simulink model "Simulink_asserv_Disc_5Avril_V2023a"  (R2023a)
settings: Solver=ode45  StartTime=0.0  StopTime=2500  FixedStep=0.01  RelTol=1e-3
model workspace (MAT data in the model file):
  AmbiantTemp = Simulink.Parameter
  AmbiantTemp.Value = 23
  AmbiantTemp.DataType = 'auto'
  AmbiantTemp.Complexity = 'real'
  AmbiantTemp.Dimensions = [1 1]
  CondSig_mesureTemp_Gain = Simulink.Parameter
  CondSig_mesureTemp_Gain.Value = 3.3
  CondSig_mesureTemp_Gain.DataType = 'auto'
  CondSig_mesureTemp_Gain.Complexity = 'real'
  CondSig_mesureTemp_Gain.Dimensions = [1 1]
  CondSig_mesureTemp_Vsub = Simulink.Parameter
  CondSig_mesureTemp_Vsub.Value = 1.85
  CondSig_mesureTemp_Vsub.DataType = 'auto'
  CondSig_mesureTemp_Vsub.Complexity = 'real'
  CondSig_mesureTemp_Vsub.Dimensions = [1 1]
  Consigne1_Temps = Simulink.Parameter
  Consigne1_Temps.Value = 640
  Consigne1_Temps.DataType = 'auto'
  Consigne1_Temps.Complexity = 'real'
  Consigne1_Temps.Dimensions = [1 1]
  Consigne1_Valeur = Simulink.Parameter
  Consigne1_Valeur.Value = 30
  Consigne1_Valeur.DataType = 'auto'
  Consigne1_Valeur.Complexity = 'real'
  Consigne1_Valeur.Dimensions = [1 1]
  Consigne2_Temps = Simulink.Parameter
  Consigne2_Temps.Value = 1290
  Consigne2_Temps.DataType = 'auto'
  Consigne2_Temps.Complexity = 'real'
  Consigne2_Temps.Dimensions = [1 1]
  Consigne2_Valeur = Simulink.Parameter
  Consigne2_Valeur.Value = 20
  Consigne2_Valeur.DataType = 'auto'
  Consigne2_Valeur.Complexity = 'real'
  Consigne2_Valeur.Dimensions = [1 1]
  Consigne3_Temps = Simulink.Parameter
  Consigne3_Temps.Value = 2130
  Consigne3_Temps.DataType = 'auto'
  Consigne3_Temps.Complexity = 'real'
  Consigne3_Temps.Dimensions = [1 1]
  Consigne3_Valeur = Simulink.Parameter
  Consigne3_Valeur.Value = 25
  Consigne3_Valeur.DataType = 'auto'
  Consigne3_Valeur.Complexity = 'real'
  Consigne3_Valeur.Dimensions = [1 1]
  DivTen_mesureTemp_R_pullup = Simulink.Parameter
  DivTen_mesureTemp_R_pullup.Value = 10000
  DivTen_mesureTemp_R_pullup.DataType = 'auto'
  DivTen_mesureTemp_R_pullup.Complexity = 'real'
  DivTen_mesureTemp_R_pullup.Dimensions = [1 1]
  DivTen_mesureTemp_Vcc = Simulink.Parameter
  DivTen_mesureTemp_Vcc.Value = 5
  DivTen_mesureTemp_Vcc.DataType = 'auto'
  DivTen_mesureTemp_Vcc.Complexity = 'real'
  DivTen_mesureTemp_Vcc.Dimensions = [1 1]
  Gain_Comparateur_VoltageControle = Simulink.Parameter
  Gain_Comparateur_VoltageControle.Value = 0.32
  Gain_Comparateur_VoltageControle.DataType = 'auto'
  Gain_Comparateur_VoltageControle.Complexity = 'real'
  Gain_Comparateur_VoltageControle.Dimensions = [1 1]
  GuT1_Denominateur = Simulink.Parameter
  GuT1_Denominateur.Value = [83.71 1]
  GuT1_Denominateur.DataType = 'auto'
  GuT1_Denominateur.Complexity = 'real'
  GuT1_Denominateur.Dimensions = [1 2]
  GuT1_Numerateur = Simulink.Parameter
  GuT1_Numerateur.Value = 9.96
  GuT1_Numerateur.DataType = 'auto'
  GuT1_Numerateur.Complexity = 'real'
  GuT1_Numerateur.Dimensions = [1 1]
  GuT2_Denominateur = Simulink.Parameter
  GuT2_Denominateur.Value = [909.26 121.79 1]
  GuT2_Denominateur.DataType = 'auto'
  GuT2_Denominateur.Complexity = 'real'
  GuT2_Denominateur.Dimensions = [1 3]
  GuT2_Numerateur = Simulink.Parameter
  GuT2_Numerateur.Value = 8.07
  GuT2_Numerateur.DataType = 'auto'
  GuT2_Numerateur.Complexity = 'real'
  GuT2_Numerateur.Dimensions = [1 1]
  GuT3_Denominateur = Simulink.Parameter
  GuT3_Denominateur.Value = [2602.39 136.94 1]
  GuT3_Denominateur.DataType = 'auto'
  GuT3_Denominateur.Complexity = 'real'
  GuT3_Denominateur.Dimensions = [1 3]
  GuT3_Numerateur = Simulink.Parameter
  GuT3_Numerateur.Value = 7.09
  GuT3_Numerateur.DataType = 'auto'
  GuT3_Numerateur.Complexity = 'real'
  GuT3_Numerateur.Dimensions = [1 1]
  Nombre_bits_ADC = Simulink.Parameter
  Nombre_bits_ADC.Value = 10
  Nombre_bits_ADC.DataType = 'auto'
  Nombre_bits_ADC.Complexity = 'real'
  Nombre_bits_ADC.Dimensions = [1 1]
  Nombre_bits_DAC = Simulink.Parameter
  Nombre_bits_DAC.Value = 8
  Nombre_bits_DAC.DataType = 'auto'
  Nombre_bits_DAC.Complexity = 'real'
  Nombre_bits_DAC.Dimensions = [1 1]
  PerturbT1_Denominateur = Simulink.Parameter
  PerturbT1_Denominateur.Value = [127 1]
  PerturbT1_Denominateur.DataType = 'auto'
  PerturbT1_Denominateur.Complexity = 'real'
  PerturbT1_Denominateur.Dimensions = [1 2]
  PerturbT1_Numerateur = Simulink.Parameter
  PerturbT1_Numerateur.Value = 20.9
  PerturbT1_Numerateur.DataType = 'auto'
  PerturbT1_Numerateur.Complexity = 'real'
  PerturbT1_Numerateur.Dimensions = [1 1]
  PerturbT2_Denominateur = Simulink.Parameter
  PerturbT2_Denominateur.Value = [144 1]
  PerturbT2_Denominateur.DataType = 'auto'
  PerturbT2_Denominateur.Complexity = 'real'
  PerturbT2_Denominateur.Dimensions = [1 2]
  PerturbT2_Numerateur = Simulink.Parameter
  PerturbT2_Numerateur.Value = 22
  PerturbT2_Numerateur.DataType = 'auto'
  PerturbT2_Numerateur.Complexity = 'real'
  PerturbT2_Numerateur.Dimensions = [1 1]
  PerturbT3_Denominateur = Simulink.Parameter
  PerturbT3_Denominateur.Value = [3300 167 1]
  PerturbT3_Denominateur.DataType = 'auto'
  PerturbT3_Denominateur.Complexity = 'real'
  PerturbT3_Denominateur.Dimensions = [1 3]
  PerturbT3_Numerateur = Simulink.Parameter
  PerturbT3_Numerateur.Value = 18.7
  PerturbT3_Numerateur.DataType = 'auto'
  PerturbT3_Numerateur.Complexity = 'real'
  PerturbT3_Numerateur.Dimensions = [1 1]
  Perturbation_Resistance = Simulink.Parameter
  Perturbation_Resistance.Value = 25
  Perturbation_Resistance.DataType = 'auto'
  Perturbation_Resistance.Complexity = 'real'
  Perturbation_Resistance.Dimensions = [1 1]
  Perturbation_TempsApplication = Simulink.Parameter
  Perturbation_TempsApplication.Value = 100
  Perturbation_TempsApplication.DataType = 'auto'
  Perturbation_TempsApplication.Complexity = 'real'
  Perturbation_TempsApplication.Dimensions = [1 1]
  Perturbation_Tension = Simulink.Parameter
  Perturbation_Tension.Value = 5
  Perturbation_Tension.DataType = 'auto'
  Perturbation_Tension.Complexity = 'real'
  Perturbation_Tension.Dimensions = [1 1]
  RC_deno = Simulink.Parameter
  RC_deno.Value = [3.22e-08 3.04e-05 0.00955 1]
  RC_deno.DataType = 'auto'
  RC_deno.Complexity = 'real'
  RC_deno.Dimensions = [1 4]
  Regulateur_Denominateur = Simulink.Parameter
  Regulateur_Denominateur.Value = [1 -1.913 0.913]
  Regulateur_Denominateur.DataType = 'auto'
  Regulateur_Denominateur.Complexity = 'real'
  Regulateur_Denominateur.Dimensions = [1 3]
  Regulateur_Numerateur = Simulink.Parameter
  Regulateur_Numerateur.Value = [1 -1.8995 0.901]
  Regulateur_Numerateur.DataType = 'auto'
  Regulateur_Numerateur.Complexity = 'real'
  Regulateur_Numerateur.Dimensions = [1 3]
  SourceCourant_Gain_Vcontrole_vers_A = Simulink.Parameter
  SourceCourant_Gain_Vcontrole_vers_A.Value = 3.1564
  SourceCourant_Gain_Vcontrole_vers_A.DataType = 'auto'
  SourceCourant_Gain_Vcontrole_vers_A.Complexity = 'real'
  SourceCourant_Gain_Vcontrole_vers_A.Dimensions = [1 1]
  T1T3_Denominateur = Simulink.Parameter
  T1T3_Denominateur.Value = [1 -1.9517 0.9522]
  T1T3_Denominateur.DataType = 'auto'
  T1T3_Denominateur.Complexity = 'real'
  T1T3_Denominateur.Dimensions = [1 3]
  T1T3_Numerateur = Simulink.Parameter
  T1T3_Numerateur.Value = [0 0.00019425 0.00019111]
  T1T3_Numerateur.DataType = 'auto'
  T1T3_Numerateur.Complexity = 'real'
  T1T3_Numerateur.Dimensions = [1 3]
  T2T3_Denominateur = Simulink.Parameter
  T2T3_Denominateur.Value = [1 -0.9655]
  T2T3_Denominateur.DataType = 'auto'
  T2T3_Denominateur.Complexity = 'real'
  T2T3_Denominateur.Dimensions = [1 2]
  T2T3_Numerateur = Simulink.Parameter
  T2T3_Numerateur.Value = [0 0.0303]
  T2T3_Numerateur.DataType = 'auto'
  T2T3_Numerateur.Complexity = 'real'
  T2T3_Numerateur.Dimensions = [1 2]
  ThermoRes_SHTEMP_A = Simulink.Parameter
  ThermoRes_SHTEMP_A.Value = 0.003354
  ThermoRes_SHTEMP_A.DataType = 'auto'
  ThermoRes_SHTEMP_A.Complexity = 'real'
  ThermoRes_SHTEMP_A.Dimensions = [1 1]
  ThermoRes_SHTEMP_B = Simulink.Parameter
  ThermoRes_SHTEMP_B.Value = 0.00026
  ThermoRes_SHTEMP_B.DataType = 'auto'
  ThermoRes_SHTEMP_B.Complexity = 'real'
  ThermoRes_SHTEMP_B.Dimensions = [1 1]
  ThermoRes_SHTEMP_C = Simulink.Parameter
  ThermoRes_SHTEMP_C.Value = 1.6e-06
  ThermoRes_SHTEMP_C.DataType = 'auto'
  ThermoRes_SHTEMP_C.Complexity = 'real'
  ThermoRes_SHTEMP_C.Dimensions = [1 1]
  ThermoRes_SHTEMP_D = Simulink.Parameter
  ThermoRes_SHTEMP_D.Value = 6.3e-08
  ThermoRes_SHTEMP_D.DataType = 'auto'
  ThermoRes_SHTEMP_D.Complexity = 'real'
  ThermoRes_SHTEMP_D.Dimensions = [1 1]
  ThermoRes_SH_A = Simulink.Parameter
  ThermoRes_SH_A.Value = -14.65719
  ThermoRes_SH_A.DataType = 'auto'
  ThermoRes_SH_A.Complexity = 'real'
  ThermoRes_SH_A.Dimensions = [1 1]
  ThermoRes_SH_B = Simulink.Parameter
  ThermoRes_SH_B.Value = 4798.842
  ThermoRes_SH_B.DataType = 'auto'
  ThermoRes_SH_B.Complexity = 'real'
  ThermoRes_SH_B.Dimensions = [1 1]
  ThermoRes_SH_C = Simulink.Parameter
  ThermoRes_SH_C.Value = -115334
  ThermoRes_SH_C.DataType = 'auto'
  ThermoRes_SH_C.Complexity = 'real'
  ThermoRes_SH_C.Dimensions = [1 1]
  ThermoRes_SH_D = Simulink.Parameter
  ThermoRes_SH_D.Value = -3730535
  ThermoRes_SH_D.DataType = 'auto'
  ThermoRes_SH_D.Complexity = 'real'
  ThermoRes_SH_D.Dimensions = [1 1]
  ThermoRes_SH_R_nom = Simulink.Parameter
  ThermoRes_SH_R_nom.Value = 10000
  ThermoRes_SH_R_nom.DataType = 'auto'
  ThermoRes_SH_R_nom.Complexity = 'real'
  ThermoRes_SH_R_nom.Dimensions = [1 1]
  periodeEchant = Simulink.Parameter
  periodeEchant.Value = 2
  periodeEchant.DataType = 'auto'
  periodeEchant.Complexity = 'real'
  periodeEchant.Dimensions = [1 1]
  periodeEchant_temp = Simulink.Parameter
  periodeEchant_temp.Value = 0.5
  periodeEchant_temp.DataType = 'auto'
  periodeEchant_temp.Complexity = 'real'
  periodeEchant_temp.Dimensions = [1 1]
  setupDelay = Simulink.Parameter
  setupDelay.Value = 4
  setupDelay.DataType = 'auto'
  setupDelay.Complexity = 'real'
  setupDelay.Dimensions = [1 1]
libraries: simulink x1
settings Model: SimulationMode=rapid-accelerator  ParameterArgumentNames=Perturbation_Resistance  Creator=alcot161  LastModifiedBy=alcot161
settings RTWCC: GPUComputeCapability=5.0

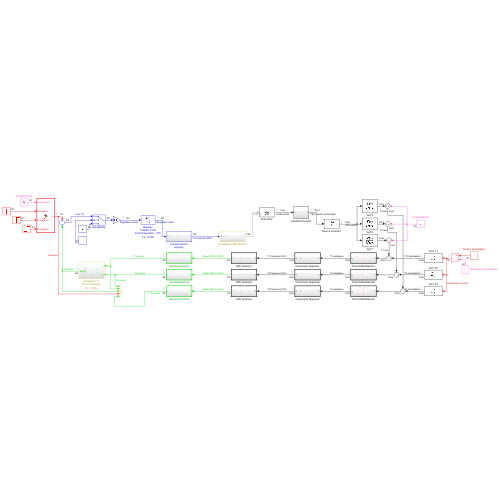
[thumbnail: Simulink's stored preview of the top-level diagram]
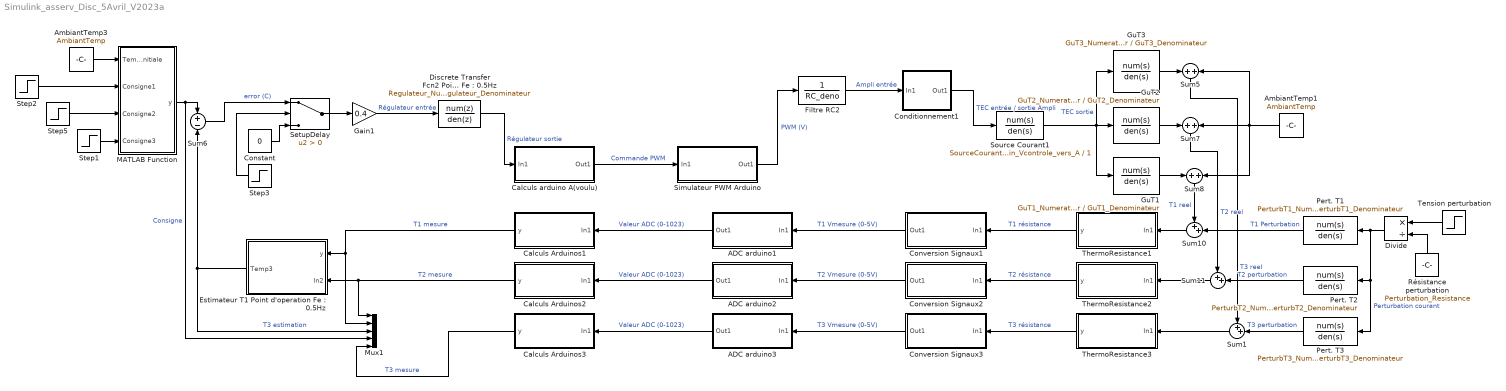
== system Simulink_asserv_Disc_5Avril_V2023a ==
  ADC arduino1 : Subsystem  TreatAsAtomicUnit=on
  ADC arduino2 : Subsystem  TreatAsAtomicUnit=on
  ADC arduino3 : Subsystem  TreatAsAtomicUnit=on
  AmbiantTemp1 : Constant  Value=AmbiantTemp
  AmbiantTemp3 : Constant  Value=AmbiantTemp
  Calculs Arduinos1 : Subsystem  TreatAsAtomicUnit=on
  Calculs Arduinos2 : Subsystem  TreatAsAtomicUnit=on
  Calculs Arduinos3 : Subsystem  TreatAsAtomicUnit=on
  "Calculs arduino A(voulu) " : Subsystem
  Conditionnement1 : Subsystem
  Constant : Constant  Value=0  SampleTime=periodeEchant
  Conversion Signaux1 : Subsystem  TreatAsAtomicUnit=on
  Conversion Signaux2 : Subsystem  TreatAsAtomicUnit=on
  Conversion Signaux3 : Subsystem  TreatAsAtomicUnit=on
  "Discrete Transfer Fcn2 Point d'operation : 27C Fe : 0.5Hz" : DiscreteTransferFcn  Numerator=Regulateur_Numerateur  Denominator=Regulateur_Denominateur
  Divide : Product  Inputs=*/
  "Estimateur T1 Point d'operation Fe : 0.5Hz" : Subsystem
  Filtre RC2 : TransferFcn  Denominator=RC_deno
  Gain1 : Gain  Gain=0.4
  GuT1 : TransferFcn  Numerator=GuT1_Numerateur  Denominator=GuT1_Denominateur
  GuT2 : TransferFcn  Numerator=GuT2_Numerateur  Denominator=GuT2_Denominateur
  GuT3 : TransferFcn  Numerator=GuT3_Numerateur  Denominator=GuT3_Denominateur
  MATLAB Function : MATLAB Function  TreatAsAtomicUnit=on
  Mux1 : Mux  Inputs=5
  Pert. T1 : TransferFcn  Numerator=PerturbT1_Numerateur  Denominator=PerturbT1_Denominateur
  Pert. T2 : TransferFcn  Numerator=PerturbT2_Numerateur  Denominator=PerturbT2_Denominateur
  Pert. T3 : TransferFcn  Numerator=PerturbT3_Numerateur  Denominator=PerturbT3_Denominateur
  Résistance perturbation : Constant  Value=Perturbation_Resistance
  SetupDelay : Switch  Criteria=u2 > Threshold  SaturateOnIntegerOverflow=off  InputSameDT=off
  Simulateur PWM Arduino : Subsystem
  Source Courant1 : TransferFcn  Numerator=SourceCourant_Gain_Vcontrole_vers_A  Denominator=1
  Step1 : Step  Time=Consigne3_Temps  After=Consigne3_Valeur  SampleTime=0.05
  Step2 : Step  Time=Consigne1_Temps  After=Consigne1_Valeur  SampleTime=0.05
  Step3 : Step  Time=setupDelay+1  SampleTime=periodeEchant
  Step5 : Step  Time=Consigne2_Temps  After=Consigne2_Valeur  SampleTime=0.05
  Sum1 : Sum  Inputs=++|
  Sum10 : Sum  Inputs=++|
  Sum11 : Sum  Inputs=++|
  Sum5 : Sum  Inputs=+|+
  Sum6 : Sum  Inputs=+|-  SampleTime=periodeEchant
  Sum7 : Sum  Inputs=+|+
  Sum8 : Sum  Inputs=+|+
  Tension perturbation : Step  Time=Perturbation_TempsApplication  After=Perturbation_Tension  SampleTime=0.05
  ThermoResistance1 : Subsystem  TreatAsAtomicUnit=on
  ThermoResistance2 : Subsystem  TreatAsAtomicUnit=on
  ThermoResistance3 : Subsystem  TreatAsAtomicUnit=on
  wires:
  ThermoResistance2/1(y) -> Conversion Signaux2/1(In1)  "T2 résistance"
  GuT2/1 -> Sum7/1
  Conversion Signaux2/1(Out1) -> ADC arduino2/1(In1)  "T2 Vmesure (0-5V)"
  ADC arduino2/1(Out1) -> Calculs Arduinos2/1(In1)  "Valeur ADC (0-1023)"
  Simulateur PWM Arduino/1(Out1) -> Filtre RC2/1  "PWM (V)"
  Step5/1 -> MATLAB Function/3(Consigne2)
  Conversion Signaux1/1(Out1) -> ADC arduino1/1(In1)  "T1 Vmesure (0-5V)"
  AmbiantTemp1/1 -> Sum5/2, Sum8/2, Sum7/2
  Filtre RC2/1 -> Conditionnement1/1(In1)  "Ampli entrée"
  Calculs Arduinos1/1(y) -> Mux1/2, "Estimateur T1 Point d'operation Fe : 0.5Hz"/1(y)  "T1 mesure"
  ADC arduino1/1(Out1) -> Calculs Arduinos1/1(In1)  "Valeur ADC (0-1023)"
  "Calculs arduino A(voulu) "/1(Out1) -> Simulateur PWM Arduino/1(In1)  "Commande PWM"
  Calculs Arduinos2/1(y) -> "Estimateur T1 Point d'operation Fe : 0.5Hz"/2(In2), Mux1/1  "T2 mesure"
  Source Courant1/1 -> GuT3/1, GuT1/1, GuT2/1  "TEC sortie"
  ThermoResistance1/1(y) -> Conversion Signaux1/1(In1)  "T1 résistance"
  Sum7/1 -> Sum11/1  "T2 reel"
  Conditionnement1/1(Out1) -> Source Courant1/1  "TEC entrée / sortie Ampli"
  GuT1/1 -> Sum8/1
  GuT3/1 -> Sum5/1
  "Discrete Transfer Fcn2 Point d'operation : 27C Fe : 0.5Hz"/1 -> "Calculs arduino A(voulu) "/1(In1)  "Régulateur sortie"
  "Estimateur T1 Point d'operation Fe : 0.5Hz"/1(Temp3) -> Sum6/2, Mux1/3  "T3 estimation"
  Step3/1 -> SetupDelay/2
  Gain1/1 -> "Discrete Transfer Fcn2 Point d'operation : 27C Fe : 0.5Hz"/1  "Régulateur entrée"
  Sum6/1 -> SetupDelay/1  "error (C)"
  SetupDelay/1 -> Gain1/1
  Constant/1 -> SetupDelay/3
  Sum8/1 -> Sum10/1  "T1 reel"
  Sum10/1 -> ThermoResistance1/1(In1)
  Sum11/1 -> ThermoResistance2/1(In1)
  Step1/1 -> MATLAB Function/4(Consigne3)
  Résistance perturbation/1 -> Divide/2
  Tension perturbation/1 -> Divide/1
  Divide/1 -> Pert. T3/1, Pert. T2/1, Pert. T1/1  "Perturbation courant"
  Pert. T1/1 -> Sum10/2  "T1 Perturbation"
  AmbiantTemp3/1 -> MATLAB Function/1(TempInitiale)
  Step2/1 -> MATLAB Function/2(Consigne1)
  MATLAB Function/1(y) -> Mux1/4, Sum6/1  "Consigne"
  Calculs Arduinos3/1(y) -> Mux1/5  "T3 mesure"
  ThermoResistance3/1(y) -> Conversion Signaux3/1(In1)  "T3 résistance"
  ADC arduino3/1(Out1) -> Calculs Arduinos3/1(In1)  "Valeur ADC (0-1023)"
  Conversion Signaux3/1(Out1) -> ADC arduino3/1(In1)  "T3 Vmesure (0-5V)"
  Sum5/1 -> Sum1/1  "T3 reel"
  Pert. T2/1 -> Sum11/2  "T2 perturbation"
  Pert. T3/1 -> Sum1/2  "T3 perturbation"
  Sum1/1 -> ThermoResistance3/1(In1)

== system Simulink_asserv_Disc_5Avril_V2023a/ADC arduino1 ==
  In1 : Inport
  Floor : Rounding
  Gain : Gain  Gain=2^Nombre_bits_ADC/5
  Out1 : Outport  SampleTime=periodeEchant_temp
  wires:
  In1/1 -> Gain/1
  Gain/1 -> Floor/1
  Floor/1 -> Out1/1

== system Simulink_asserv_Disc_5Avril_V2023a/ADC arduino2 ==
  In1 : Inport
  Floor : Rounding
  Gain : Gain  Gain=2^Nombre_bits_ADC/5
  Out1 : Outport  SampleTime=periodeEchant_temp
  wires:
  In1/1 -> Gain/1
  Gain/1 -> Floor/1
  Floor/1 -> Out1/1

== system Simulink_asserv_Disc_5Avril_V2023a/ADC arduino3 ==
  In1 : Inport
  Floor : Rounding
  Gain : Gain  Gain=2^Nombre_bits_ADC/5
  Out1 : Outport  SampleTime=periodeEchant_temp
  wires:
  In1/1 -> Gain/1
  Gain/1 -> Floor/1
  Floor/1 -> Out1/1

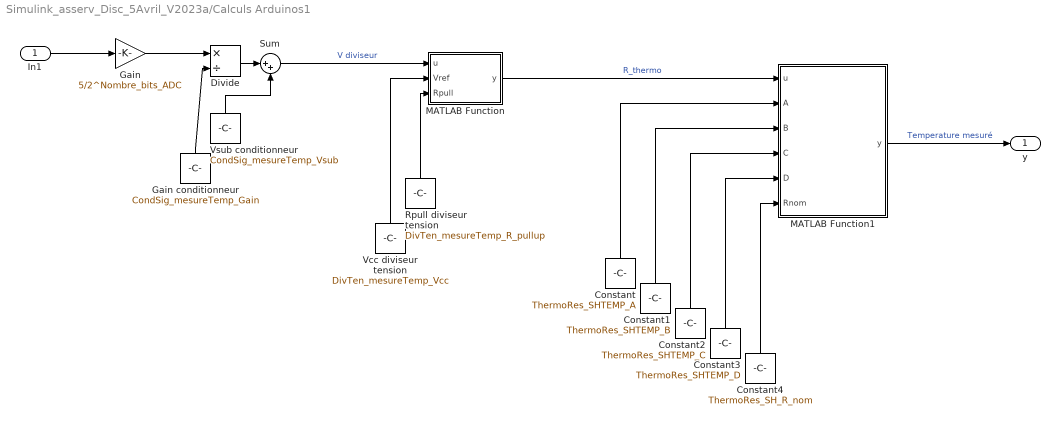
== system Simulink_asserv_Disc_5Avril_V2023a/Calculs Arduinos1 ==
  In1 : Inport
  Constant : Constant  Value=ThermoRes_SHTEMP_A
  Constant1 : Constant  Value=ThermoRes_SHTEMP_B
  Constant2 : Constant  Value=ThermoRes_SHTEMP_C
  Constant3 : Constant  Value=ThermoRes_SHTEMP_D
  Constant4 : Constant  Value=ThermoRes_SH_R_nom
  Divide : Product  Inputs=*/
  Gain : Gain  Gain=5/2^Nombre_bits_ADC
  Gain conditionneur : Constant  Value=CondSig_mesureTemp_Gain
  MATLAB Function : MATLAB Function  TreatAsAtomicUnit=on
  MATLAB Function1 : MATLAB Function  TreatAsAtomicUnit=on
  Rpull diviseur tension : Constant  Value=DivTen_mesureTemp_R_pullup
  Sum : Sum  Inputs=|++
  Vcc diviseur tension : Constant  Value=DivTen_mesureTemp_Vcc
  Vsub conditionneur : Constant  Value=CondSig_mesureTemp_Vsub
  y : Outport
  wires:
  In1/1 -> Gain/1
  Gain/1 -> Divide/1
  Gain conditionneur/1 -> Divide/2
  Divide/1 -> Sum/1
  Vsub conditionneur/1 -> Sum/2
  Sum/1 -> MATLAB Function/1(u)  "V diviseur"
  Rpull diviseur tension/1 -> MATLAB Function/3(Rpull)
  Vcc diviseur tension/1 -> MATLAB Function/2(Vref)
  MATLAB Function/1(y) -> MATLAB Function1/1(u)  "R_thermo"
  Constant/1 -> MATLAB Function1/2(A)
  Constant1/1 -> MATLAB Function1/3(B)
  Constant2/1 -> MATLAB Function1/4(C)
  Constant3/1 -> MATLAB Function1/5(D)
  Constant4/1 -> MATLAB Function1/6(Rnom)
  MATLAB Function1/1(y) -> y/1  "Temperature mesuré"

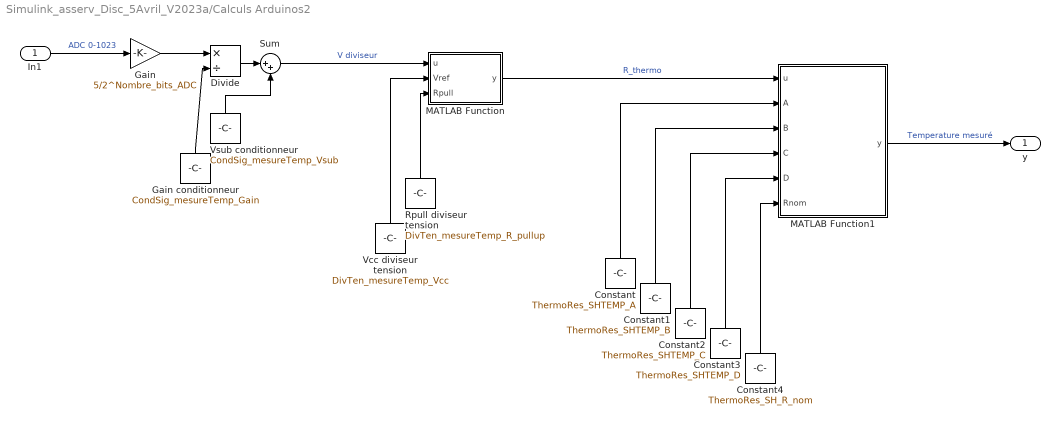
== system Simulink_asserv_Disc_5Avril_V2023a/Calculs Arduinos2 ==
  In1 : Inport
  Constant : Constant  Value=ThermoRes_SHTEMP_A
  Constant1 : Constant  Value=ThermoRes_SHTEMP_B
  Constant2 : Constant  Value=ThermoRes_SHTEMP_C
  Constant3 : Constant  Value=ThermoRes_SHTEMP_D
  Constant4 : Constant  Value=ThermoRes_SH_R_nom
  Divide : Product  Inputs=*/
  Gain : Gain  Gain=5/2^Nombre_bits_ADC
  Gain conditionneur : Constant  Value=CondSig_mesureTemp_Gain
  MATLAB Function : MATLAB Function  TreatAsAtomicUnit=on
  MATLAB Function1 : MATLAB Function  TreatAsAtomicUnit=on
  Rpull diviseur tension : Constant  Value=DivTen_mesureTemp_R_pullup
  Sum : Sum  Inputs=|++
  Vcc diviseur tension : Constant  Value=DivTen_mesureTemp_Vcc
  Vsub conditionneur : Constant  Value=CondSig_mesureTemp_Vsub
  y : Outport
  wires:
  In1/1 -> Gain/1  "ADC 0-1023"
  Gain/1 -> Divide/1
  Gain conditionneur/1 -> Divide/2
  Divide/1 -> Sum/1
  Vsub conditionneur/1 -> Sum/2
  Sum/1 -> MATLAB Function/1(u)  "V diviseur"
  Rpull diviseur tension/1 -> MATLAB Function/3(Rpull)
  Vcc diviseur tension/1 -> MATLAB Function/2(Vref)
  MATLAB Function/1(y) -> MATLAB Function1/1(u)  "R_thermo"
  Constant/1 -> MATLAB Function1/2(A)
  Constant1/1 -> MATLAB Function1/3(B)
  Constant2/1 -> MATLAB Function1/4(C)
  Constant3/1 -> MATLAB Function1/5(D)
  Constant4/1 -> MATLAB Function1/6(Rnom)
  MATLAB Function1/1(y) -> y/1  "Temperature mesuré"

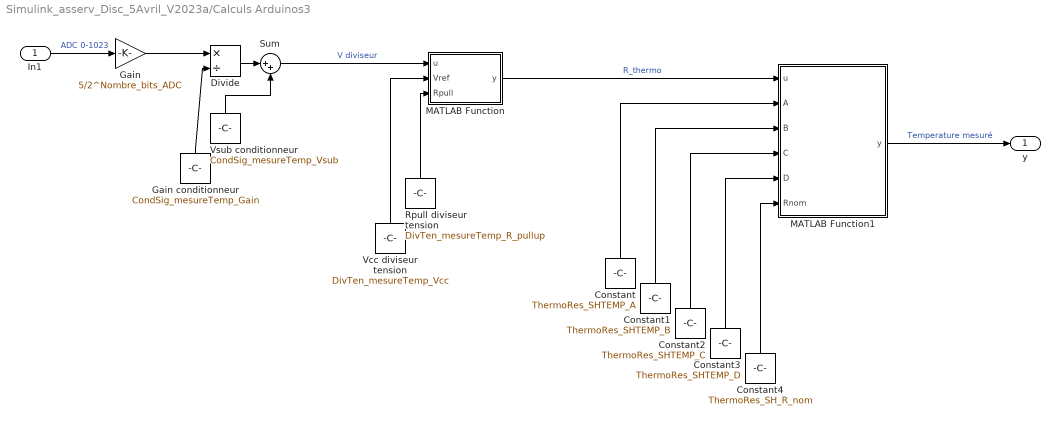
== system Simulink_asserv_Disc_5Avril_V2023a/Calculs Arduinos3 ==
  In1 : Inport
  Constant : Constant  Value=ThermoRes_SHTEMP_A
  Constant1 : Constant  Value=ThermoRes_SHTEMP_B
  Constant2 : Constant  Value=ThermoRes_SHTEMP_C
  Constant3 : Constant  Value=ThermoRes_SHTEMP_D
  Constant4 : Constant  Value=ThermoRes_SH_R_nom
  Divide : Product  Inputs=*/
  Gain : Gain  Gain=5/2^Nombre_bits_ADC
  Gain conditionneur : Constant  Value=CondSig_mesureTemp_Gain
  MATLAB Function : MATLAB Function  TreatAsAtomicUnit=on
  MATLAB Function1 : MATLAB Function  TreatAsAtomicUnit=on
  Rpull diviseur tension : Constant  Value=DivTen_mesureTemp_R_pullup
  Sum : Sum  Inputs=|++
  Vcc diviseur tension : Constant  Value=DivTen_mesureTemp_Vcc
  Vsub conditionneur : Constant  Value=CondSig_mesureTemp_Vsub
  y : Outport
  wires:
  In1/1 -> Gain/1  "ADC 0-1023"
  Gain/1 -> Divide/1
  Gain conditionneur/1 -> Divide/2
  Divide/1 -> Sum/1
  Vsub conditionneur/1 -> Sum/2
  Sum/1 -> MATLAB Function/1(u)  "V diviseur"
  Rpull diviseur tension/1 -> MATLAB Function/3(Rpull)
  Vcc diviseur tension/1 -> MATLAB Function/2(Vref)
  MATLAB Function/1(y) -> MATLAB Function1/1(u)  "R_thermo"
  Constant/1 -> MATLAB Function1/2(A)
  Constant1/1 -> MATLAB Function1/3(B)
  Constant2/1 -> MATLAB Function1/4(C)
  Constant3/1 -> MATLAB Function1/5(D)
  Constant4/1 -> MATLAB Function1/6(Rnom)
  MATLAB Function1/1(y) -> y/1  "Temperature mesuré"

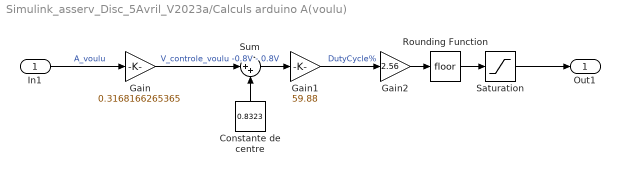
== system Simulink_asserv_Disc_5Avril_V2023a/Calculs arduino A(voulu)  ==
  In1 : Inport
  Constante de centre : Constant  Value=0.8323
  Gain : Gain  Gain=0.3168166265365
  Gain1 : Gain  Gain=59.88
  Gain2 : Gain  Gain=2.56  ParamMin=0  ParamMax=255.9  OutMin=[0]  OutMax=[255]
  Rounding Function : Rounding
  Saturation : Saturate  UpperLimit=2^Nombre_bits_DAC-1  LowerLimit=0  LinearizeAsGain=off
  Sum : Sum  Inputs=|++
  Out1 : Outport
  wires:
  In1/1 -> Gain/1  "A_voulu"
  Gain/1 -> Sum/1  "V_controle_voulu -0.8V - 0.8V"
  Sum/1 -> Gain1/1
  Constante de centre/1 -> Sum/2
  Gain1/1 -> Gain2/1  "DutyCycle%"
  Gain2/1 -> Rounding Function/1
  Rounding Function/1 -> Saturation/1
  Saturation/1 -> Out1/1

== system Simulink_asserv_Disc_5Avril_V2023a/Conditionnement1 ==
  In1 : Inport
  Constant : Constant  Value=2.5
  Gain : Gain  Gain=Gain_Comparateur_VoltageControle
  Subtract : Sum  Inputs=+-
  Out1 : Outport
  wires:
  In1/1 -> Subtract/1
  Constant/1 -> Subtract/2
  Subtract/1 -> Gain/1
  Gain/1 -> Out1/1

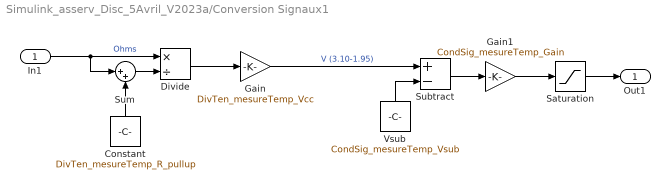
== system Simulink_asserv_Disc_5Avril_V2023a/Conversion Signaux1 ==
  In1 : Inport
  Constant : Constant  Value=DivTen_mesureTemp_R_pullup
  Divide : Product  Inputs=*/
  Gain : Gain  Gain=DivTen_mesureTemp_Vcc
  Gain1 : Gain  Gain=CondSig_mesureTemp_Gain
  Saturation : Saturate  UpperLimit=5  LowerLimit=0
  Subtract : Sum  Inputs=+-
  Sum : Sum  Inputs=|++
  Vsub : Constant  Value=CondSig_mesureTemp_Vsub
  Out1 : Outport
  wires:
  In1/1 -> Sum/1, Divide/1  "Ohms"
  Sum/1 -> Divide/2
  Constant/1 -> Sum/2
  Divide/1 -> Gain/1
  Vsub/1 -> Subtract/2
  Subtract/1 -> Gain1/1
  Gain1/1 -> Saturation/1
  Saturation/1 -> Out1/1
  Gain/1 -> Subtract/1  "V (3.10-1.95)"

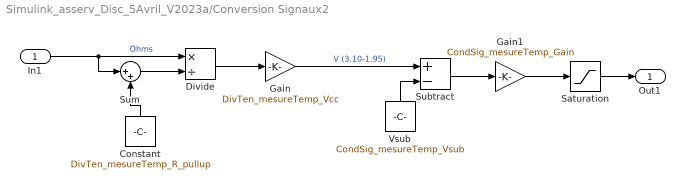
== system Simulink_asserv_Disc_5Avril_V2023a/Conversion Signaux2 ==
  In1 : Inport
  Constant : Constant  Value=DivTen_mesureTemp_R_pullup
  Divide : Product  Inputs=*/
  Gain : Gain  Gain=DivTen_mesureTemp_Vcc
  Gain1 : Gain  Gain=CondSig_mesureTemp_Gain
  Saturation : Saturate  UpperLimit=5  LowerLimit=0
  Subtract : Sum  Inputs=+-
  Sum : Sum  Inputs=|++
  Vsub : Constant  Value=CondSig_mesureTemp_Vsub
  Out1 : Outport
  wires:
  In1/1 -> Sum/1, Divide/1  "Ohms"
  Sum/1 -> Divide/2
  Constant/1 -> Sum/2
  Divide/1 -> Gain/1
  Vsub/1 -> Subtract/2
  Subtract/1 -> Gain1/1
  Gain1/1 -> Saturation/1
  Saturation/1 -> Out1/1
  Gain/1 -> Subtract/1  "V (3.10-1.95)"

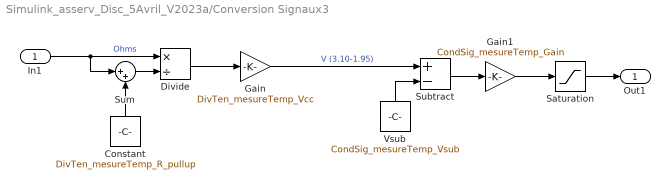
== system Simulink_asserv_Disc_5Avril_V2023a/Conversion Signaux3 ==
  In1 : Inport
  Constant : Constant  Value=DivTen_mesureTemp_R_pullup
  Divide : Product  Inputs=*/
  Gain : Gain  Gain=DivTen_mesureTemp_Vcc
  Gain1 : Gain  Gain=CondSig_mesureTemp_Gain
  Saturation : Saturate  UpperLimit=5  LowerLimit=0
  Subtract : Sum  Inputs=+-
  Sum : Sum  Inputs=|++
  Vsub : Constant  Value=CondSig_mesureTemp_Vsub
  Out1 : Outport
  wires:
  In1/1 -> Sum/1, Divide/1  "Ohms"
  Sum/1 -> Divide/2
  Constant/1 -> Sum/2
  Divide/1 -> Gain/1
  Vsub/1 -> Subtract/2
  Subtract/1 -> Gain1/1
  Gain1/1 -> Saturation/1
  Saturation/1 -> Out1/1
  Gain/1 -> Subtract/1  "V (3.10-1.95)"

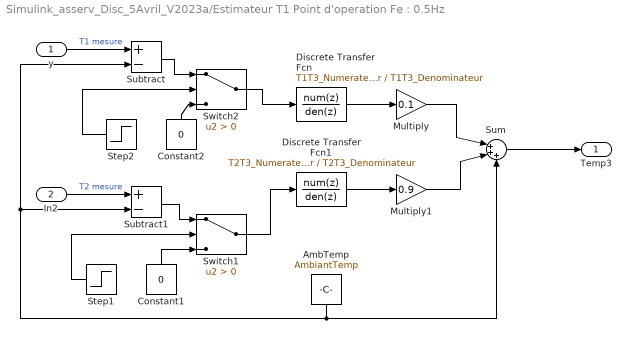
== system Simulink_asserv_Disc_5Avril_V2023a/Estimateur T1 Point d'operation Fe : 0.5Hz ==
  y : Inport
  In2 : Inport  Port=2
  AmbTemp : Constant  Value=AmbiantTemp  SampleTime=periodeEchant_temp
  Constant1 : Constant  Value=0  SampleTime=2
  Constant2 : Constant  Value=0  SampleTime=2
  Discrete Transfer Fcn : DiscreteTransferFcn  Numerator=T1T3_Numerateur  Denominator=T1T3_Denominateur
  Discrete Transfer Fcn1 : DiscreteTransferFcn  Numerator=T2T3_Numerateur  Denominator=T2T3_Denominateur
  Multiply : Gain  Gain=0.1
  Multiply1 : Gain  Gain=0.9
  Step1 : Step  Time=setupDelay  SampleTime=periodeEchant
  Step2 : Step  Time=setupDelay  SampleTime=periodeEchant
  Subtract : Sum  Inputs=+-
  Subtract1 : Sum  Inputs=+-
  Sum : Sum  Inputs=|+++
  Switch1 : Switch  Criteria=u2 > Threshold  SaturateOnIntegerOverflow=off  InputSameDT=off
  Switch2 : Switch  Criteria=u2 > Threshold  SaturateOnIntegerOverflow=off  InputSameDT=off
  Temp3 : Outport  SampleTime=periodeEchant_temp
  wires:
  In2/1 -> Subtract1/1  "T2 mesure"
  Multiply/1 -> Sum/1
  Multiply1/1 -> Sum/2
  y/1 -> Subtract/1  "T1 mesure"
  Sum/1 -> Temp3/1
  Discrete Transfer Fcn/1 -> Multiply/1
  Discrete Transfer Fcn1/1 -> Multiply1/1
  AmbTemp/1 -> Subtract/2, Subtract1/2, Sum/3
  Constant1/1 -> Switch1/3
  Constant2/1 -> Switch2/3
  Step2/1 -> Switch2/2
  Subtract/1 -> Switch2/1
  Switch2/1 -> Discrete Transfer Fcn/1
  Subtract1/1 -> Switch1/1
  Step1/1 -> Switch1/2
  Switch1/1 -> Discrete Transfer Fcn1/1

== system Simulink_asserv_Disc_5Avril_V2023a/Simulateur PWM Arduino ==
  In1 : Inport
  Gain1 : Gain  Gain=1/((2^Nombre_bits_DAC)-1)
  Gain2 : Gain  Gain=5
  PWM : simulink/Discontinuities/PWM  DisableCoverage=on  Period=0.00204  InitialDelay=0  DisallowZeroDutyCycle=off  RunAtFixedTimeIntervals=off  SampleTime=0.1
  Out1 : Outport
  wires:
  Gain1/1 -> PWM/1
  PWM/1 -> Gain2/1  "PWM / DAC sortie"
  In1/1 -> Gain1/1
  Gain2/1 -> Out1/1

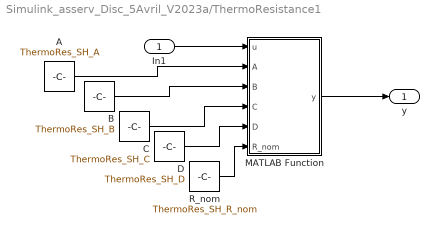
== system Simulink_asserv_Disc_5Avril_V2023a/ThermoResistance1 ==
  In1 : Inport
  A : Constant  Value=ThermoRes_SH_A
  B : Constant  Value=ThermoRes_SH_B
  C : Constant  Value=ThermoRes_SH_C
  D : Constant  Value=ThermoRes_SH_D
  MATLAB Function : MATLAB Function  TreatAsAtomicUnit=on
  R_nom : Constant  Value=ThermoRes_SH_R_nom
  y : Outport
  wires:
  In1/1 -> MATLAB Function/1(u)
  MATLAB Function/1(y) -> y/1
  A/1 -> MATLAB Function/2(A)
  B/1 -> MATLAB Function/3(B)
  C/1 -> MATLAB Function/4(C)
  D/1 -> MATLAB Function/5(D)
  R_nom/1 -> MATLAB Function/6(R_nom)

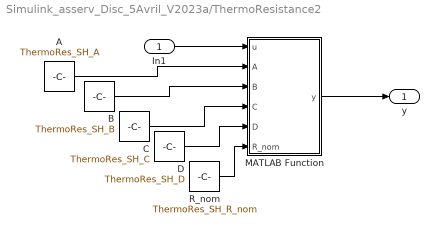
== system Simulink_asserv_Disc_5Avril_V2023a/ThermoResistance2 ==
  In1 : Inport
  A : Constant  Value=ThermoRes_SH_A
  B : Constant  Value=ThermoRes_SH_B
  C : Constant  Value=ThermoRes_SH_C
  D : Constant  Value=ThermoRes_SH_D
  MATLAB Function : MATLAB Function  TreatAsAtomicUnit=on
  R_nom : Constant  Value=ThermoRes_SH_R_nom
  y : Outport
  wires:
  In1/1 -> MATLAB Function/1(u)
  MATLAB Function/1(y) -> y/1
  A/1 -> MATLAB Function/2(A)
  B/1 -> MATLAB Function/3(B)
  C/1 -> MATLAB Function/4(C)
  D/1 -> MATLAB Function/5(D)
  R_nom/1 -> MATLAB Function/6(R_nom)

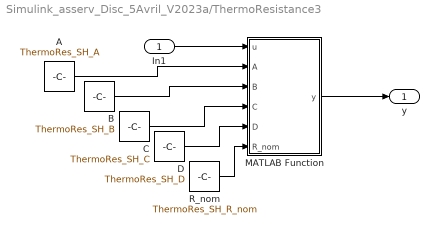
== system Simulink_asserv_Disc_5Avril_V2023a/ThermoResistance3 ==
  In1 : Inport
  A : Constant  Value=ThermoRes_SH_A
  B : Constant  Value=ThermoRes_SH_B
  C : Constant  Value=ThermoRes_SH_C
  D : Constant  Value=ThermoRes_SH_D
  MATLAB Function : MATLAB Function  TreatAsAtomicUnit=on
  R_nom : Constant  Value=ThermoRes_SH_R_nom
  y : Outport
  wires:
  In1/1 -> MATLAB Function/1(u)
  MATLAB Function/1(y) -> y/1
  A/1 -> MATLAB Function/2(A)
  B/1 -> MATLAB Function/3(B)
  C/1 -> MATLAB Function/4(C)
  D/1 -> MATLAB Function/5(D)
  R_nom/1 -> MATLAB Function/6(R_nom)

== matlab function Simulink_asserv_Disc_5Avril_V2023a/ThermoResistance2/MATLAB Function ==
  data: u input; y output; A input; B input; C input; D input; R_nom input
function y = fcn(u, A, B, C, D, R_nom)
   
y = R_nom * exp(A + (B/(u+273.15)) + (C/((u + 273.15)^2)) + (D/((u + 273.15)^3)));

== matlab function Simulink_asserv_Disc_5Avril_V2023a/MATLAB Function ==
  data: TempInitiale input; y output; Consigne1 input; Consigne2 input; Consigne3 input
function y = fcn(TempInitiale, Consigne1, Consigne2, Consigne3)
   
y = TempInitiale;
if (Consigne1 ~= 0)
    y = Consigne1;
end
if (Consigne2 ~= 0)
    y = Consigne2;
end
if (Consigne3 ~= 0)
    y = Consigne3;
end
if (y > 30)
    y = 30;
end
if (y < 20)
    y = 20;
end

== matlab function Simulink_asserv_Disc_5Avril_V2023a/Calculs Arduinos3/MATLAB Function ==
  data: u input; y output; Vref input; Rpull input
function y = fcn(u, Vref, Rpull)

y = Rpull * (u/(Vref-u));

== matlab function Simulink_asserv_Disc_5Avril_V2023a/Calculs Arduinos3/MATLAB Function1 ==
  data: u input; y output; A input; B input; C input; D input; Rnom input
function y = fcn(u, A, B, C, D, Rnom)
    invT = A + B*log(u/Rnom) + C*(log(u/Rnom))^2 + D*(log(u/Rnom))^3;
    T = (1/invT) - 273.15;
y = T;

== matlab function Simulink_asserv_Disc_5Avril_V2023a/ThermoResistance3/MATLAB Function ==
  data: u input; y output; A input; B input; C input; D input; R_nom input
function y = fcn(u, A, B, C, D, R_nom)
   
y = R_nom * exp(A + (B/(u+273.15)) + (C/((u + 273.15)^2)) + (D/((u + 273.15)^3)));

== matlab function Simulink_asserv_Disc_5Avril_V2023a/Calculs Arduinos1/MATLAB Function ==
  data: u input; y output; Vref input; Rpull input
function y = fcn(u, Vref, Rpull)

y = Rpull * (u/(Vref-u));

== matlab function Simulink_asserv_Disc_5Avril_V2023a/Calculs Arduinos1/MATLAB Function1 ==
  data: u input; y output; A input; B input; C input; D input; Rnom input
function y = fcn(u, A, B, C, D, Rnom)
    invT = A + B*log(u/Rnom) + C*(log(u/Rnom))^2 + D*(log(u/Rnom))^3;
    T = (1/invT) - 273.15;
y = T;

== matlab function Simulink_asserv_Disc_5Avril_V2023a/Calculs Arduinos2/MATLAB Function ==
  data: u input; y output; Vref input; Rpull input
function y = fcn(u, Vref, Rpull)

y = Rpull * (u/(Vref-u));

== matlab function Simulink_asserv_Disc_5Avril_V2023a/Calculs Arduinos2/MATLAB Function1 ==
  data: u input; y output; A input; B input; C input; D input; Rnom input
function y = fcn(u, A, B, C, D, Rnom)
    invT = A + B*log(u/Rnom) + C*(log(u/Rnom))^2 + D*(log(u/Rnom))^3;
    T = (1/invT) - 273.15;
y = T;

== matlab function Simulink_asserv_Disc_5Avril_V2023a/ThermoResistance1/MATLAB Function ==
  data: u input; y output; A input; B input; C input; D input; R_nom input
function y = fcn(u, A, B, C, D, R_nom)
   
y = R_nom * exp(A + (B/(u+273.15)) + (C/((u + 273.15)^2)) + (D/((u + 273.15)^3)));
